simulink library "thrustVectorControl_cl"  (R2020a)
settings: Solver=VariableStepAuto  StartTime=0.0  StopTime=10.0  RelTol=1e-3
settings Model: Creator=jbore  LastModifiedBy=John Jr
settings SFSimCC: CustomCodeUndefinedFunction=UseInterfaceOnly

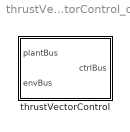
== system thrustVectorControl_cl ==
  thrustVectorControl : Subsystem

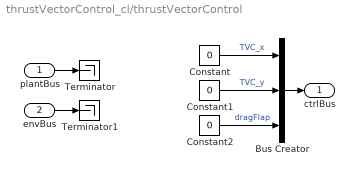
== system thrustVectorControl_cl/thrustVectorControl ==
  plantBus : Inport
  envBus : Inport  Port=2
  Bus Creator : BusCreator  Inputs=3
  Constant : Constant  Value=0
  Constant1 : Constant  Value=0
  Constant2 : Constant  Value=0
  Terminator : Terminator
  Terminator1 : Terminator
  ctrlBus : Outport  VectorParamsAs1DForOutWhenUnconnected=off
  wires:
  Bus Creator/1 -> ctrlBus/1
  plantBus/1 -> Terminator/1
  envBus/1 -> Terminator1/1
  Constant/1 -> Bus Creator/1  "TVC_x"
  Constant1/1 -> Bus Creator/2  "TVC_y"
  Constant2/1 -> Bus Creator/3  "dragFlap"
